simulink model "Chap6_ComplexBaseband"  (R2015a)
settings: Solver=VariableStepDiscrete  StartTime=0.0  StopTime=10  RelTol=1e-3
InitFcn:
  | clear
  | M = 16;
  | l = log2(M);
  | SNR = 10;
  | EsN0 = SNR;
  | EbN0 = SNR - 10 * log10(l);
  | BERTheory = berawgn(EbN0, 'qam', M);
libraries: commdigbbndam3 x5, commchan3 x4, commsink2 x4, commrandsrc2 x1
settings Model: Creator=Administrator  LastModifiedBy=Administrator
settings DebuggingCC: SignalRangeChecking=warning  ParameterOverflowMsg=warning  ParameterPrecisionLossMsg=none  ParameterTunabilityLossMsg=none
settings HardwareCC: ProdHWDeviceType=ASIC/FPGA->ASIC/FPGA  TargetHWDeviceType=Generic->Custom  ProdEqTarget=off

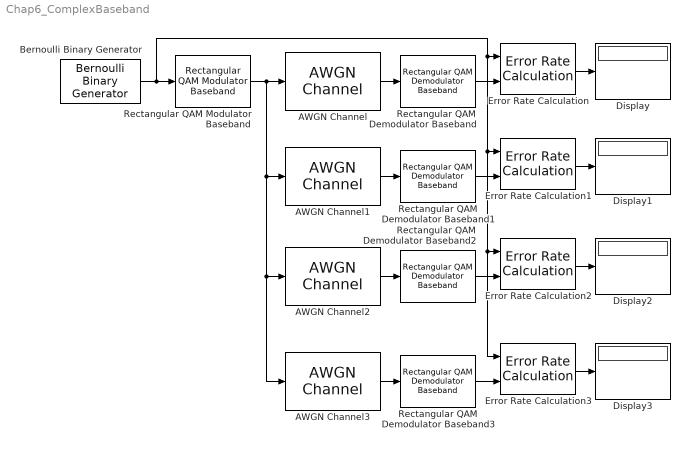
== system Chap6_ComplexBaseband ==
  AWGN Channel : commchan3/AWGN Channel  InputProcessing=Columns as channels (frame based)  seed=67  noiseMode="Signal to noise ratio  (SNR)"  EbNodB=10  EsNodB=10  SNRdB=SNR  bitsPerSym=4  Ps=1  Tsym=4e-6  variance=1
  AWGN Channel1 : commchan3/AWGN Channel  InputProcessing=Columns as channels (frame based)  seed=67  noiseMode="Signal to noise ratio  (Es/No)"  EbNodB=10  EsNodB=EsN0  SNRdB=10  bitsPerSym=1  Ps=1  Tsym=4e-6  variance=1
  AWGN Channel2 : commchan3/AWGN Channel  InputProcessing=Columns as channels (frame based)  seed=67  noiseMode="Signal to noise ratio  (Eb/No)"  EbNodB=EbN0  EsNodB=10  SNRdB=15 - 10*log10(4)  bitsPerSym=4  Ps=1  Tsym=4e-6  variance=1
  AWGN Channel3 : commchan3/AWGN Channel  InputProcessing=Columns as channels (frame based)  seed=67  noiseMode=Variance from mask  EbNodB=10  EsNodB=10  SNRdB=1  bitsPerSym=1  Ps=1  Tsym=1  variance=1 / (10^(SNR/10))
  Bernoulli Binary Generator : commrandsrc2/Bernoulli Binary Generator  P=0.5  seed=61  Ts=1e-6  frameBased=on  sampPerFrame=4  orient=off  outDataType=double
  Display{,1..3} (4 alike) : Display
  Error Rate Calculation{,1..3} (4 alike) : commsink2/Error Rate Calculation  N=0  st_delay=0  cp_mode=Entire frame  subframe=[]  PMode=Port  WsName=ErrorVec  RsMode2=off  stop=off  numErr=100  maxBits=1e6
  Rectangular QAM Demodulator Baseband{,1..3} (4 alike) : commdigbbndam3/Rectangular QAM Demodulator Baseband  M=16  PowType=Average Power  MinDist=2  AvgPow=1  PeakPow=1  Ph=0  Dec=Gray  Mapping=[0:15]  OutType=Bit  DecType=Hard decision  VarSource=Dialog  Variance=1  outDtype1=Inherit via internal rule  outDtype2=Inherit via internal rule  derotateFactorWordLen=16  denormFactorWordLen=16  prodOutWordLen=32  prodOutRoundingMode=Floor  prodOutOverflowMode=Wrap  sumWordLen=32
  Rectangular QAM Modulator Baseband : commdigbbndam3/Rectangular QAM Modulator Baseband  M=16  InType=Bit  Enc=Gray  Mapping=[0:15]  PowType=Average Power  MinDist=2  AvgPow=1  PeakPow=1  Ph=0  outDtype=double  outWordLen=16  outUDDataType=sfix(16)  outFracLenMode=Best precision  outFracLen=15
  wires:
  Bernoulli Binary Generator/1 -> Error Rate Calculation/1, Error Rate Calculation1/1, Error Rate Calculation2/1, Error Rate Calculation3/1, Rectangular QAM Modulator Baseband/1
  Rectangular QAM Modulator Baseband/1 -> AWGN Channel/1, AWGN Channel2/1, AWGN Channel3/1, AWGN Channel1/1
  AWGN Channel/1 -> Rectangular QAM Demodulator Baseband/1
  AWGN Channel1/1 -> Rectangular QAM Demodulator Baseband1/1
  AWGN Channel2/1 -> Rectangular QAM Demodulator Baseband2/1
  Rectangular QAM Demodulator Baseband/1 -> Error Rate Calculation/2
  Rectangular QAM Demodulator Baseband1/1 -> Error Rate Calculation1/2
  Rectangular QAM Demodulator Baseband2/1 -> Error Rate Calculation2/2
  Error Rate Calculation1/1 -> Display1/1
  Error Rate Calculation2/1 -> Display2/1
  Error Rate Calculation/1 -> Display/1
  AWGN Channel3/1 -> Rectangular QAM Demodulator Baseband3/1
  Rectangular QAM Demodulator Baseband3/1 -> Error Rate Calculation3/2
  Error Rate Calculation3/1 -> Display3/1
